simulink model "ECBtn_DD"  (R2016b)
settings: configuration reference "CodeGenConfigSet" (kept outside this file)
values from neighbouring files (symbols this model uses):
  ECBtn_stStopReplVal_C = Calibration.Parameter    [init_ECBtn_DD.m]    (also in init_ECBtn_DD_SIL.m = Simulink.Parameter)
  ECBtn_stStrtReplVal_C = Calibration.Parameter    [init_ECBtn_DD.m]    (also in init_ECBtn_DD_SIL.m = Simulink.Parameter)
  ECBtn_swtSigSelStop_C = Calibration.Parameter    [init_ECBtn_DD.m]    (also in init_ECBtn_DD_SIL.m = Simulink.Parameter)
  ECBtn_swtSigSelStrt_C = Calibration.Parameter    [init_ECBtn_DD.m]    (also in init_ECBtn_DD_SIL.m = Simulink.Parameter)
  ECBtn_tiStopDebHiLo_C = Calibration.Parameter    [init_ECBtn_DD.m]    (also in init_ECBtn_DD_SIL.m = Simulink.Parameter)
  ECBtn_tiStopDebLoHi_C = Calibration.Parameter    [init_ECBtn_DD.m]    (also in init_ECBtn_DD_SIL.m = Simulink.Parameter)
  ECBtn_tiStrtDebHiLo_C = Calibration.Parameter    [init_ECBtn_DD.m]    (also in init_ECBtn_DD_SIL.m = Simulink.Parameter)
  ECBtn_tiStrtDebLoHi_C = Calibration.Parameter    [init_ECBtn_DD.m]    (also in init_ECBtn_DD_SIL.m = Simulink.Parameter)
undefined symbols (not defined in the file or in its folder): ECBtn_DD_DT
libraries: CXLib x2
settings Model: Creator=xinchangran  LastModifiedBy=xinchangran
settings ConfigSetRef: SourceLocation=Base Workspace

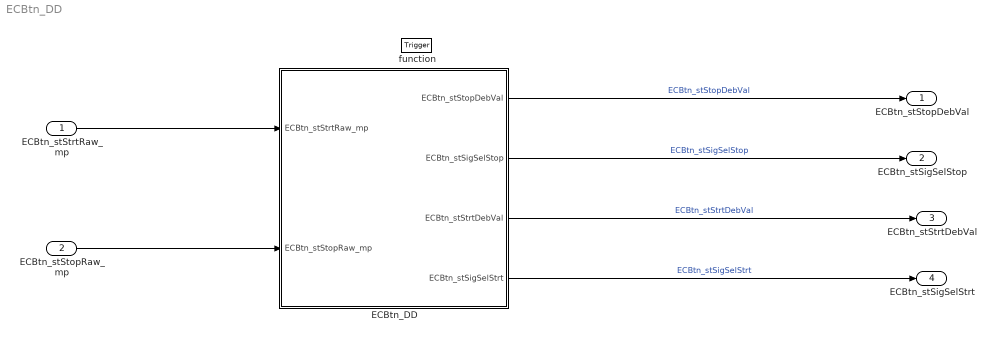
== system ECBtn_DD ==
  ECBtn_stStrtRaw_mp : Inport  Description=start state  OutMin=0  OutMax=1  OutDataTypeStr=boolean
  ECBtn_stStopRaw_mp : Inport  Description=stop state  Port=2  OutMin=0  OutMax=1  OutDataTypeStr=boolean
  function : TriggerPort  TriggerType=function-call  VariantControl=Variant
  ECBtn_DD : Subsystem
  ECBtn_stStopDebVal : Outport  Description=stop signal  OutMin=0  OutMax=1  OutDataTypeStr=boolean
  ECBtn_stSigSelStop : Outport  Description=Calibration stop signal  Port=2  OutMin=0  OutMax=1  OutDataTypeStr=boolean
  ECBtn_stStrtDebVal : Outport  Description=start signal  Port=3  OutMin=0  OutMax=1  OutDataTypeStr=boolean
  ECBtn_stSigSelStrt : Outport  Description=Calibration start signal  Port=4  OutMin=0  OutMax=1  OutDataTypeStr=boolean
  wires:
  ECBtn_stStrtRaw_mp/1 -> ECBtn_DD/1(ECBtn_stStrtRaw_mp)
  ECBtn_stStopRaw_mp/1 -> ECBtn_DD/2(ECBtn_stStopRaw_mp)
  ECBtn_DD/1(ECBtn_stStopDebVal) -> ECBtn_stStopDebVal/1  "ECBtn_stStopDebVal"
  ECBtn_DD/2(ECBtn_stSigSelStop) -> ECBtn_stSigSelStop/1  "ECBtn_stSigSelStop"
  ECBtn_DD/3(ECBtn_stStrtDebVal) -> ECBtn_stStrtDebVal/1  "ECBtn_stStrtDebVal"
  ECBtn_DD/4(ECBtn_stSigSelStrt) -> ECBtn_stSigSelStrt/1  "ECBtn_stSigSelStrt"

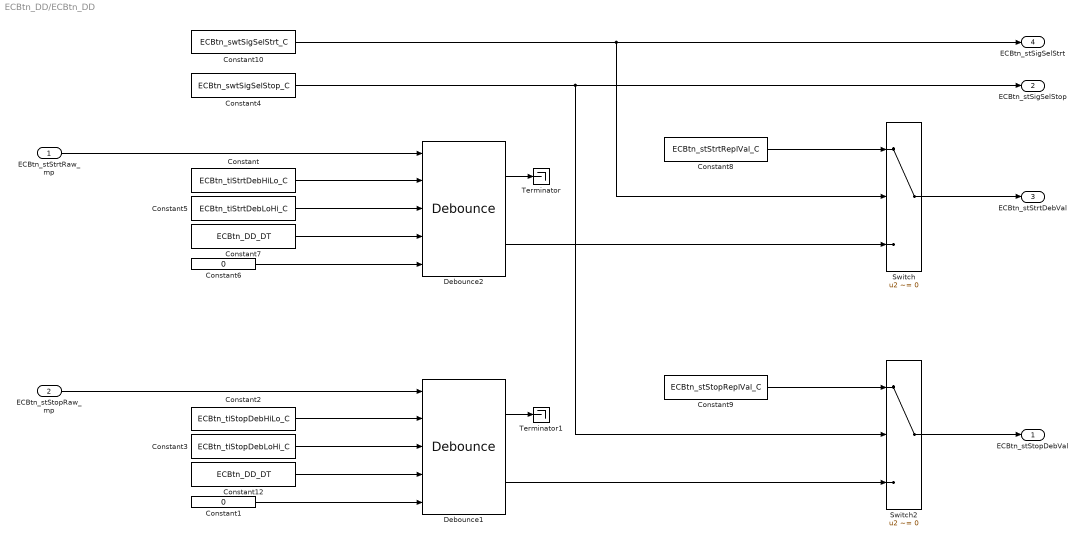
== system ECBtn_DD/ECBtn_DD ==
  ECBtn_stStrtRaw_mp : Inport  Description=start state  OutMin=0  OutMax=1  OutDataTypeStr=boolean
  ECBtn_stStopRaw_mp : Inport  Description=stop state  Port=2  OutMin=0  OutMax=1  OutDataTypeStr=boolean
  Constant : Constant  Value=ECBtn_tiStrtDebHiLo_C
  Constant1 : Constant  Value=0  OutDataTypeStr=Inherit: Inherit via back propagation
  Constant10 : Constant  Value=ECBtn_swtSigSelStrt_C  SampleTime=-1
  Constant12 : Constant  Value=ECBtn_DD_DT
  Constant2 : Constant  Value=ECBtn_tiStopDebHiLo_C
  Constant3 : Constant  Value=ECBtn_tiStopDebLoHi_C
  Constant4 : Constant  Value=ECBtn_swtSigSelStop_C  SampleTime=-1
  Constant5 : Constant  Value=ECBtn_tiStrtDebLoHi_C
  Constant6 : Constant  Value=0  OutDataTypeStr=Inherit: Inherit via back propagation
  Constant7 : Constant  Value=ECBtn_DD_DT
  Constant8 : Constant  Value=ECBtn_stStrtReplVal_C
  Constant9 : Constant  Value=ECBtn_stStopReplVal_C
  Debounce1 : CXLib/Debounce
  Debounce2 : CXLib/Debounce
  Switch : Switch  Criteria=u2 ~= 0  InputSameDT=on
  Switch2 : Switch  Criteria=u2 ~= 0  InputSameDT=on
  Terminator : Terminator
  Terminator1 : Terminator
  ECBtn_stStopDebVal : Outport  Description=stop signal  OutMin=0  OutMax=1  OutDataTypeStr=boolean
  ECBtn_stSigSelStop : Outport  Description=Calibration stop signal  Port=2  OutMin=0  OutMax=1
  ECBtn_stStrtDebVal : Outport  Description=start signal  Port=3  OutMin=0  OutMax=1  OutDataTypeStr=boolean
  ECBtn_stSigSelStrt : Outport  Description=Calibration start signal  Port=4  OutMin=0  OutMax=1
  wires:
  Switch/1 -> ECBtn_stStrtDebVal/1
  Constant5/1 -> Debounce2/3
  Constant7/1 -> Debounce2/4
  Constant6/1 -> Debounce2/5
  Constant/1 -> Debounce2/2
  Debounce2/2 -> Switch/3
  Debounce2/1 -> Terminator/1
  Constant8/1 -> Switch/1
  Constant3/1 -> Debounce1/3
  Constant12/1 -> Debounce1/4
  Constant1/1 -> Debounce1/5
  Constant2/1 -> Debounce1/2
  Debounce1/1 -> Terminator1/1
  ECBtn_stStrtRaw_mp/1 -> Debounce2/1
  ECBtn_stStopRaw_mp/1 -> Debounce1/1
  Constant10/1 -> Switch/2, ECBtn_stSigSelStrt/1
  Debounce1/2 -> Switch2/3
  Constant9/1 -> Switch2/1
  Constant4/1 -> Switch2/2, ECBtn_stSigSelStop/1
  Switch2/1 -> ECBtn_stStopDebVal/1
